simulink library "carnot"  (R2018b)
settings: Solver=VariableStepAuto  StartTime=0.0  StopTime=10.0  RelTol=1e-3
undefined symbols (not defined in the file or in its folder): A, A_earth, acol, Acol, ActPower1, ActPower2, ActPower3, Ad, Ad0, Ar, Au, Au0, Azimuth_Angle, B, Bd, Bd0, Br, Bu, Bu0, C, c1, c2, c3, c33, c4, c5, c6, CarnotCallbacks_Density, CarnotCallbacks_Enthalpy, CarnotCallbacks_Enthalpy2Temperature, CarnotCallbacks_Entropy, CarnotCallbacks_Evaporation_Enthalpy, CarnotCallbacks_GlobalMessageLevel, CarnotCallbacks_Grashof, CarnotCallbacks_Heat_Capacity, CarnotCallbacks_Kinematic_Viscosity, CarnotCallbacks_PMV_PPD, CarnotCallbacks_Prandtl, CarnotCallbacks_Saturation_Property, CarnotCallbacks_Saturation_Temperature, CarnotCallbacks_Saturation_Value_Water, CarnotCallbacks_Specific_Volume, CarnotCallbacks_Thermal_Conductivity, CarnotCallbacks_Vapour_Content, CarnotCallbacks_Vapour_Pressure, Cd, Cdl, Cr, Cu, Davies, Dd, DE_TRY2010_04_averageYear, delta_grd, density, DiameterLastPiece, dl, DPConstant, DPLinear, DPQuadratic, Dr ... (+59)
libraries: $bdroot x429, simulink x36, simulink_extras x12
(part 16 of 22)

== system carnot/Source/Cogeneration/microCHP_modulating ==
  THBreturn_load : Inport
  control : Inport  Port=2
  Bus Creator : BusCreator  Inputs=8
  Constant : Constant  Value=f_P_el
  Control_Unit : Subsystem
  Demux : Demux  Outputs=[1 1 1 1 1 1]
  Demux3 : Demux  Outputs=[6 14]
  Ground : Ground
  Heat_Capacity : $bdroot/Basic/Material_Properties/Heat_Capacity  VariantControl=CarlibClassic  INPUTARGUMENTS=state variables (classic)  DEBUGLEVEL=DEBUGLEVEL  MAXTOTALWARNINGS=inf  MAXCONSECUTIVEWARNINGS=inf  WRITETOFILE=0  FILENAME='errors.txt'
  Mux1 : Mux  Inputs=[1 1 1 1 1 1 14]
  Product : Product  Inputs=//*  SaturateOnIntegerOverflow=on  RndMeth=Zero  InputSameDT=on  OutDataTypeStr=Inherit: Same as first input
  Product1 : Product  Inputs=**  SaturateOnIntegerOverflow=on  RndMeth=Zero  InputSameDT=on  OutDataTypeStr=Inherit: Same as first input
  Product2 : Product  Inputs=**  SaturateOnIntegerOverflow=on  RndMeth=Zero  InputSameDT=on  OutDataTypeStr=Inherit: Same as first input
  Storage_Type_0 : $bdroot/Storage/Thermal/Storage_Type_0  t0=25  hgt=0.95493  stgtype=0  mpts=[1 2 3 4 5]  tini=[25 25 25 25 25]  PathName=fullfile(path_carnot('libsl'),'Storage','Thermal','Storage_Type_0','parameter_set')  FileName='<user defined>'  userPath=off  userParam=on  uwall=1  ubot=1  utop=1  axcond=1  volume=0.03  dia=0.2  standing=standing cylinder  nodes=5  mpoints=5  Tsensor=0.5  pipe1inlet=1  pipe1outlet=0  pipe1dia=0.03  heater1start=0.2  heater1end=0.25
  Sum : Sum  SaturateOnIntegerOverflow=on  InputSameDT=on  OutDataTypeStr=Inherit: Same as first input
  THB2THV : $bdroot/Toolbox/THB2THV
  THB2THV1 : $bdroot/Toolbox/THB2THV
  THV2THB : $bdroot/Toolbox/THV2THB
  THV2THB1 : $bdroot/Toolbox/THV2THB
  T_Sensor : $bdroot/Control/T_Sensor  tc=10  t0=20
  T_amb : Constant  Value=15
  Terminator : Terminator
  Terminator1 : Terminator
  energy and efficiency : Subsystem
  f_P_gas_lookup-table : Lookup_n-D  NumberOfTableDimensions=1  BreakpointsForDimension1=[1,2]  BreakpointsForDimension2=[44,80]  BreakpointsForDimension3=[1:2]  BreakpointsForDimension4=[1:2]  Table=[1.79 1.5]  InputSameDT=on
  measure_T : Subsystem  mask(temperature measurement sensor){tc=10, t0=25}
      mask prompts: tc "time constant of sensor [s]"; t0 "initial temperature [degree centigrade]"
      mask help: Measurement sensor for temperatures with first-oder hold. Temperature is in degree centigrade.
      mask init:
      | tc = 1/max(tc, 0.001);
      mask Help: eval('man (''measure_T'')')
      mask Display: plot(-18,0,30,20,[0 20],[0 0],[10 10 8 8 12 12 10],[0 8 8 17 17 8 8],[10 10 9 9 11 11 10 9],[15 10 10 9 9 10 9 10])
  measure_mdot : Subsystem  mask(massflow measurement sensor){}
      mask help: Measurement sensor for massflow in kg/s.
      mask Help: eval('man (''measure_mdot'')')
  pump_const : Subsystem  mask(constant pump){mdotmax=0.3, fluid_id=water, mix=0, dia=0.0157, power=100, p0=3e5}
      mask prompts: mdotmax "massflow rate [kg/s]"; fluid_id "fluid"; mix "percentage of fluid mix [0..1]"; dia "diameter at in- and outlet [m]"; power "electric power consumption [W]"; p0 "system pressure [Pa]"
      mask help: set constant massflow rate
      mask init:
      | mix = min(1, max(0, mix));
      | dia = max(0.001, dia);
      | p0 = max(p0, 1e5);
      mask Help: eval('man(''pump_const'')')
      mask TypeOptions fluid_id: water | air | cotton_oil | silicone_oil | water_glycol_mix
      mask Display: plot(0,0,100,100,[40,70,40,30,30,40,60,70,70,60,40],[70,50,30,40,60,70,70,60,40,30,30])
  return temperature raising facility : Subsystem  mask(return temperature raising facility){}
      mask help: A return setpoint temperature is calculated depending on heating power and flow setpoint temperature. The thermostatic mixer is located in the return flow of the CHP.
  scale_function : Subsystem
  zeroavoiding : Saturate  UpperLimit=inf  LowerLimit=1e-5
  THBflow_load : Outport
  data : Outport  Port=2
  wires:
  Ground/1 -> Storage_Type_0/3
  THBreturn_load/1 -> T_Sensor/1
  T_Sensor/2 -> Control_Unit/5(T_return_load)
  Storage_Type_0/2 -> Terminator1/1
  Demux/4 -> Mux1/4, Heat_Capacity/2  "p"
  Demux/1 -> Mux1/1  "ID"
  Demux/5 -> Mux1/5, Heat_Capacity/3
  Demux/6 -> Mux1/6, Heat_Capacity/4
  Demux/3 -> Mux1/3, zeroavoiding/1  "mdot"
  Sum/1 -> Mux1/2
  Demux3/1 -> Demux/1
  Demux3/2 -> Mux1/7
  Mux1/1 -> THV2THB1/1
  Product/1 -> Sum/2
  Demux/2 -> Heat_Capacity/1, Sum/1  "T"
  Heat_Capacity/1 -> Control_Unit/1(cp), Product/2
  measure_T/1(T) -> Control_Unit/3(T_flow)
  measure_mdot/2(mdot) -> Control_Unit/2(mdot_return)
  zeroavoiding/1 -> Product/1
  THB2THV1/1 -> pump_const/1(THVin)
  pump_const/1(THV) -> measure_T/1(THV_in)
  Control_Unit/1(control_CHP) -> Bus Creator/7, pump_const/2(control), energy and efficiency/1(control CHP)  "ControlActual"
  Control_Unit/2(P_th) -> Product/3, return temperature raising facility/2(P_th), energy and efficiency/2(P_th), Product2/1, scale_function/1(P_th), Product1/1
  scale_function/1(X_pth) -> f_P_gas_lookup-table/1
  Product2/1 -> energy and efficiency/4(P_el)
  f_P_gas_lookup-table/1 -> Product1/2
  Product1/1 -> energy and efficiency/3(P_gas)
  return temperature raising facility/1(THB_return) -> THB2THV/1
  measure_T/2(THV) -> THV2THB/1
  measure_mdot/1(THV) -> Demux3/1
  Constant/1 -> Product2/2
  energy and efficiency/1(Q_th) -> Bus Creator/1  "Q_th"
  energy and efficiency/2(Q_el) -> Bus Creator/2  "Q_el"
  energy and efficiency/3(Q_gas) -> Bus Creator/3  "Q_Gas"
  energy and efficiency/4(eta_th) -> Bus Creator/4  "eta_th"
  energy and efficiency/5(eta_el) -> Bus Creator/5  "eta_el"
  energy and efficiency/6(eta_sys) -> Bus Creator/6  "eta_sys"
  Bus Creator/1 -> data/1
  return temperature raising facility/2(THB_flow_load) -> THBflow_load/1
  T_Sensor/1 -> return temperature raising facility/3(THB_return_load)
  control/1 -> Bus Creator/8, Control_Unit/4(demand_control)  "ControlSetpoint"
  THB2THV/1 -> measure_mdot/1(THV_in)
  THV2THB/1 -> return temperature raising facility/1(THB_flow)
  THV2THB1/1 -> Storage_Type_0/2
  Storage_Type_0/3 -> THB2THV1/1
  T_amb/1 -> Storage_Type_0/1
  Storage_Type_0/1 -> Terminator/1

== system carnot/Source/Electric_Generator/Inverter ==
  note: power curtailment:
      | maximal possible power - actual power
  EB_DC : Inport
  P_max_set : Inport  Port=2
  1-D Lookup Table : Lookup_n-D  NumberOfTableDimensions=1  BreakpointsForDimension1=PstepsEta  Table=Eta  RndMeth=Simplest  InputSameDT=on
  Add : Sum  Inputs=+-
  Bus Assignment : BusAssignment  AssignedSignals=Frequency,Voltage1,ActPower1,Voltage2,ActPower2,Voltage3,ActPower3
  Bus Creator2 : BusCreator  Inputs=5
  Bus Selector : BusSelector  OutputSignals=ActPower1
  Compare To Zero : simulink/Logic and Bit Operations/Compare To Zero  relop===  OutDataTypeStr=boolean
  Demux : Demux  Outputs=3
  Frequency : Constant  Value=f
  Matrix1phase : Gain  Gain=[1 0 0]
  Matrix3phase : Gain  Gain=[1/3 1/3 1/3]
  MinMax : MinMax  Inputs=2
  NormialPower : Constant  Value=Pacnom
  Nphase : Constant  Value=nphase  mask{nphase=1-phase}
      mask prompts: nphase "Number of phases"
      mask TypeOptions nphase: 1-phase | 3-phase
  P_standby : Constant  Value=P_standby
  Product : Product
  Product1 : Product  Inputs=*/
  Product3 : Product
  Signal Conversion : SignalConversion  OverrideOpt=off
  Sum : Sum  Inputs=-+
  Switch : Switch  Criteria=u2 > Threshold  Threshold=1.5
  Voltage : Constant  Value=U
  basic_EB : $bdroot/Basic/Electric/basic_EB  eID=Power only  f=50  v1=230  p1=0  pf1=1  v2=230  p2=0  pf2=1  v3=230  p3=0  pf3=1
  limit_0_1 : Saturate  UpperLimit=inf  LowerLimit=0
  limit_Pacnom : Saturate  UpperLimit=Pacnom  LowerLimit=0
  only_positive : Saturate  UpperLimit=inf  LowerLimit=0
  EB_AC : Outport
  InvDat : Outport  Port=2
  wires:
  limit_Pacnom/1 -> MinMax/1, Sum/2
  limit_0_1/1 -> 1-D Lookup Table/1
  Nphase/1 -> Switch/2
  Matrix3phase/1 -> Switch/1
  Matrix1phase/1 -> Switch/3
  Switch/1 -> Demux/1
  Demux/1 -> Bus Assignment/4
  Demux/3 -> Bus Assignment/8
  Demux/2 -> Bus Assignment/6
  Voltage/1 -> Bus Assignment/3, Bus Assignment/5, Bus Assignment/7
  Frequency/1 -> Bus Assignment/2
  Bus Assignment/1 -> EB_AC/1
  basic_EB/1 -> Bus Assignment/1
  Add/1 -> Bus Creator2/1, Matrix1phase/1, Matrix3phase/1  "P_AC"
  Product3/1 -> Add/2
  P_standby/1 -> Product3/2
  Signal Conversion/1 -> Product3/1
  Compare To Zero/1 -> Signal Conversion/1
  1-D Lookup Table/1 -> Product/1
  Product/1 -> limit_Pacnom/1
  only_positive/1 -> MinMax/2
  NormialPower/1 -> Product1/2, Bus Creator2/4  "P_peak"
  Product1/1 -> limit_0_1/1
  Sum/1 -> Bus Creator2/5  "P_curtailment"
  Bus Creator2/1 -> InvDat/1  "InvDat"
  MinMax/1 -> Sum/1, Compare To Zero/1, Add/1  "P_AC"
  P_max_set/1 -> Bus Creator2/3, only_positive/1  "P_max_set"
  EB_DC/1 -> Bus Selector/1  "P_DC"
  Bus Selector/1 -> Product/2, Bus Creator2/2, Product1/1  "<ActPower1>"

== system carnot/Source/Electric_Generator/Inverter_SPI ==
  EB_PV : Inport
  EB_Load : Inport  Port=2
  PwrTarget : Inport  Port=3  Unit=W
  ac_charge_on : Inport  Port=4  Unit=W
  Bus Assignment : BusAssignment  AssignedSignals=ActPower1,ActPower2,ActPower3
  Bus Creator : BusCreator  Inputs=11
  Bus Selector : BusSelector  OutputSignals=ActPower1  OutputAsBus=on
  Bus Selector1 : BusSelector  OutputSignals=ActPower1  OutputAsBus=on
  Demux : Demux  Outputs=8
  Demux1 : Demux  Outputs=3
  Matrix1phase : Gain  Gain=[1 0 0]
  Matrix3phase : Gain  Gain=[1/3 1/3 1/3]
  Mux2 : Mux
  Nphase : Constant  Value=nphase  mask{nphase=3-phase}
      mask prompts: nphase "Number of phases"
      mask TypeOptions nphase: 1-phase | 3-phase
  S-Function : S-Function  FunctionName=Inverter_SPI  Parameters=soc0,cap_user,soc_min,soc_max,spi_data, inv_Ts  SFunctionDeploymentMode=off  EnableBusSupport=off  mask{spi_data=SpiData, soc0=soc0, soc_min=socMin, soc_max=socMax, inv_Ts=Tsample, cap_user=capUser}
      mask prompts: spi_data "SPI Parameters"; soc0 "initial state of charge"; soc_min "minimum  state of charge"; soc_max "maximum state of charge"; inv_Ts "sample Time"; cap_user "override battery capacity"
      mask init:
      | if isempty(spi_data)
      |    spi_data = [5;5;4;4;4;5;0;0;0;0;0;0;0;0;0;0;0;0;0;0;0;0;0;0;0.980000000000000;2;5;0;0;0;0;1;5;90] 
      | end
      | if isempty(soc0)
      |    soc0 = 0;
      | end
      | if isempty(soc_min)
      |    soc_min = 0;
      | end
      | if isempty(soc_max)
      |    soc_max = 0;
      | end
      | if isempty(inv_Ts)
      |    inv_Ts = 1;
      | end
      | if isempty(cap_user)
      |    cap_user = 0;
      | end
  Switch : Switch  Criteria=u2 > Threshold  Threshold=1.5
  gain : Gain  Gain=-1
  InvDat : Outport
  EB_AC : Outport  Port=2
  wires:
  EB_PV/1 -> Bus Selector/1  "P_DC"
  Demux/8 -> Bus Creator/8  "Ebat"
  Demux/2 -> Bus Creator/2  "Ppv2ac"
  Mux2/1 -> S-Function/1
  Demux/3 -> Bus Creator/3  "Pbat2ac"
  PwrTarget/1 -> Mux2/3, Bus Creator/9  "PowerTarget"
  Demux/6 -> Bus Creator/6  "Pbat"
  Demux/4 -> Bus Creator/4  "Pac2bat"
  Demux/7 -> Bus Creator/7  "SOC"
  gain/1 -> Mux2/2  "Pac"
  Demux/5 -> Bus Creator/5  "Ppv2bat"
  Bus Creator/1 -> InvDat/1
  Bus Selector/1 -> Bus Creator/10, Mux2/1  "Ppv"
  Demux/1 -> Bus Creator/1, Matrix3phase/1, Matrix1phase/1  "Ppvbs"
  S-Function/1 -> Demux/1
  EB_Load/1 -> Bus Selector1/1, Bus Assignment/1  "P_AC"
  Demux1/1 -> Bus Assignment/2
  Demux1/2 -> Bus Assignment/3
  Bus Assignment/1 -> EB_AC/1
  Demux1/3 -> Bus Assignment/4
  Nphase/1 -> Switch/2
  Matrix3phase/1 -> Switch/1
  Matrix1phase/1 -> Switch/3
  Switch/1 -> Demux1/1
  Bus Selector1/1 -> gain/1, Bus Creator/11  "Pload"
  ac_charge_on/1 -> Mux2/4

== system carnot/Source/Electric_Generator/PV_Generator ==
  WDB : Inport
  position : Inport  Port=2
  1/(1000W/m²) : Gain  Gain=1/1000
  Bus Creator : BusCreator  Inputs=4
  Bus Selector1 : BusSelector  OutputSignals=Temperature_Ambient
  EBCreator : $bdroot/Basic/Electric/EBCreator  Inport_ID=off  Inport_f=off  Inport_v1=off  Inport_p1=on  Inport_pf1=off  Inport_v2=off  Inport_p2=off  Inport_pf2=off  Inport_v3=off  Inport_p3=off  Inport_pf3=off  ID=1  f=0  v1=0  p1=1e5  pf1=1  v2=0  p2=0  pf2=0  v3=0  p3=0  pf3=0  Annotation_ID=off  Annotation_f=off  Annotation_v1=off  Annotation_p1=off  Annotation_pf1=off  Annotation_v2=off  Annotation_p2=off  Annotation_pf2=off  Annotation_v3=off  Annotation_p3=off  Annotation_pf3=off
  IAM_Table1 : $bdroot/Source/Solar_Thermal/IncidenceAngleModifier/IAM_Table  fta=1  angle=[0:5:90]  Kb="[1.0000    1.0000    0.9999    0.9996    0.9991    0.9982    0.9965  0.9935    0.9886    0.9807    0.9678    0.9473    0.9148    0.8638   0.7846    0.6644    0.4907    0.2599    0.0000]"  Kd=0.915
  Product : Product  RndMeth=Zero
  Radiation_on_Inclined_Surface : $bdroot/Weather/Radiation_on_Inclined_Surface  sky=Hay-Davies  reflect=0.2
  Sum : Sum  Inputs=-+
  T module : Sum  Inputs=2
  T0 : Constant  Value=25
  Wp : Constant  Value=Wp
  Wp_act : Sum
  delta_Wp : Product  RndMeth=Zero
  delta_Wp/K : Gain  Gain=delta_Wp_K
  factor for generator : Gain  Gain=fgen
  overheating 40K@1000W/m2 : Gain  Gain=40
  EB_power : Outport
  PVdat : Outport  Port=2
  wires:
  EBCreator/1 -> EB_power/1
  Bus Creator/1 -> PVdat/1
  delta_Wp/1 -> Wp_act/1
  Wp/1 -> delta_Wp/2, Bus Creator/4, Wp_act/2  "P_peak_PV"
  Bus Selector1/1 -> T module/2  "<Temperature_Ambient>"
  overheating 40K@1000W/m2/1 -> T module/1
  Sum/1 -> delta_Wp/K/1
  T0/1 -> Sum/2
  IAM_Table1/1 -> 1/(1000W/m²)/1
  T module/1 -> Bus Creator/3, Sum/1  "Tcell"
  Wp_act/1 -> Product/2
  1/(1000W/m²)/1 -> overheating 40K@1000W/m2/1, Product/1
  Product/1 -> factor for generator/1
  delta_Wp/K/1 -> delta_Wp/1
  factor for generator/1 -> Bus Creator/1, EBCreator/1  "P_DC"
  WDB/1 -> Bus Selector1/1, Radiation_on_Inclined_Surface/1
  Radiation_on_Inclined_Surface/1 -> IAM_Table1/1
  position/1 -> Radiation_on_Inclined_Surface/2
  IAM_Table1/2 -> Bus Creator/2  "SolarRadiaton_global_surface"

== system carnot/Source/Energy/Fuel ==
  Bus Creator : BusCreator  Inputs=13
  Demux : Demux  Outputs=6
  airdemand : Constant  Value=stoichAir
  enthalpy : Constant  Value=combustion_enthalpy
  fuel_type : Constant  Value=ft
  mass : Constant  Value=massfraction
  pressure : Constant  Value=Pressure
  price : Constant  Value=price
  tc : Constant  Value=Tcondensation
  temperature : Constant  Value=Temperature
  fuel : Outport
  wires:
  mass/1 -> Demux/1
  airdemand/1 -> Bus Creator/3  "Stoichiometric_Air_Demand"
  Demux/6 -> Bus Creator/13  "MassFraction_H2O"
  pressure/1 -> Bus Creator/4  "Pressure"
  price/1 -> Bus Creator/7  "Price"
  Demux/3 -> Bus Creator/10  "MassFraction_O"
  enthalpy/1 -> Bus Creator/5  "h_Vector"
  Demux/1 -> Bus Creator/8  "MassFraction_H"
  Bus Creator/1 -> fuel/1
  Demux/4 -> Bus Creator/11  "MassFraction_S"
  Demux/5 -> Bus Creator/12  "MassFraction_N"
  tc/1 -> Bus Creator/6  "T_h_Vector"
  fuel_type/1 -> Bus Creator/1  "Fuel_ID"
  Demux/2 -> Bus Creator/9  "MassFraction_C"
  temperature/1 -> Bus Creator/2  "Temperature"

== system carnot/Source/Heat_Exchanger/Floorheating_TABS ==
  note: source: Koschenz, M.; Lehmann, B.: Thermoaktive Bauteilsysteme tabs. EMPA, Dübendorf, 2000. ISBN 3-905594-19-6
  T(P) : Inport
  THBin : Inport  Port=2
  Bus Assignment : BusAssignment  AssignedSignals=Temperature
  Bus Selector : BusSelector  OutputSignals=Temperature,MassFlow,Pressure,FluidType,FluidMix
  Demux2 : Demux  Outputs=2
  Mux2 : Mux  Inputs=6
  S-Function : S-Function  FunctionName=tabs  Parameters=d d1 d_pipe dr dx l lambda_r lambda_b  SFunctionDeploymentMode=off  EnableBusSupport=off
  power : Outport
  THBout : Outport  Port=2  InitialOutput=0
  wires:
  T(P)/1 -> Mux2/6
  THBin/1 -> Bus Assignment/1, Bus Selector/1
  Bus Selector/4 -> Mux2/4  "<FluidType>"
  Bus Selector/3 -> Mux2/3  "<Pressure>"
  Bus Selector/2 -> Mux2/2  "<MassFlow>"
  Bus Selector/5 -> Mux2/5  "<FluidMix>"
  Bus Selector/1 -> Mux2/1  "<Temperature>"
  Mux2/1 -> S-Function/1
  S-Function/1 -> Demux2/1
  Demux2/2 -> Bus Assignment/2  "Temperature"
  Demux2/1 -> power/1
  Bus Assignment/1 -> THBout/1

== system carnot/Source/Heat_Exchanger/HeatExchanger ==
  Tamb : Inport
  THB_pri : Inport  Port=2
  THB_sec : Inport  Port=3
  Bus Assignment : BusAssignment  AssignedSignals=Temperature
  Bus Assignment1 : BusAssignment  AssignedSignals=Temperature
  Bus Selector : BusSelector  OutputSignals=Temperature,MassFlow,Pressure,FluidType,FluidMix  OutputAsBus=on
  Bus Selector1 : BusSelector  OutputSignals=Temperature,MassFlow,Pressure,FluidType,FluidMix  OutputAsBus=on
  Pressure_Drop_Fix : $bdroot/Basic/Pressure_Drop/Pressure_Drop_Fix  con=0  lin=linh  qua=quah
  Pressure_Drop_Fix1 : $bdroot/Basic/Pressure_Drop/Pressure_Drop_Fix  con=0  lin=linc  qua=quac
  S-Function : S-Function  FunctionName=heatexch  Parameters=flowtype, ua0, uahot(1), uahot(2), uacold(1), uacold(2), ualoss, cap, t0  SFunctionDeploymentMode=off  EnableBusSupport=off
  Terminator : Terminator
  THBpri : Outport
  THBsec : Outport  Port=2
  wires:
  Pressure_Drop_Fix1/1 -> THBsec/1
  Pressure_Drop_Fix/1 -> THBpri/1
  Bus Assignment1/1 -> Pressure_Drop_Fix1/1
  S-Function/2 -> Bus Assignment1/2
  Bus Assignment/1 -> Pressure_Drop_Fix/1
  S-Function/1 -> Bus Assignment/2
  Bus Selector1/1 -> S-Function/3
  THB_sec/1 -> Bus Assignment1/1, Bus Selector1/1
  THB_pri/1 -> Bus Assignment/1, Bus Selector/1
  S-Function/3 -> Terminator/1
  Bus Selector/1 -> S-Function/2
  Tamb/1 -> S-Function/1

== system carnot/Source/Heat_Exchanger/Radiator ==
  Troom : Inport
  THBin : Inport  Port=2
  Radiator_basic : $bdroot/Basic/Thermal_Models/Radiator_basic  pnomEN=pnom  dtnomEN=dtnom  expo=expo  mcp=mcap  tini=tini
  pressdrop_fix_THB : $bdroot/Basic/Pressure_Drop/Pressure_Drop_Fix  con=0  lin=lin  qua=qua
  Qdot : Outport
  THBout : Outport  Port=2
  wires:
  pressdrop_fix_THB/1 -> THBout/1
  Radiator_basic/1 -> pressdrop_fix_THB/1
  THBin/1 -> Radiator_basic/1
  Troom/1 -> Radiator_basic/2
  Radiator_basic/2 -> Qdot/1

== system carnot/Source/Heat_Exchanger/Radiator_AIV ==
  AIV : Inport
  THB_in : Inport  Port=2
  Ground : Ground
  Ground1 : Ground
  Ground2 : Ground
  Matrix Gain : Gain  Gain=[co; ra]  Multiplication=Matrix(K*u)  SaturateOnIntegerOverflow=on  OutDataTypeStr=Inherit: Same as input  ParamDataTypeStr=Inherit: Same as input
  Mux2 : Mux  Inputs=[4 1 1 2 5]
  Radiator : $bdroot/Source/Heat_Exchanger/Radiator  pnom=pnom  dtnom=dtnom  expo=expo  mcap=mcap  tini=tini  lin=lin  qua=qua
  Troom : Subsystem
  S : Outport
  THB_out : Outport  Port=2
  wires:
  Ground/1 -> Mux2/1
  Ground2/1 -> Mux2/3
  Ground1/1 -> Mux2/5
  Mux2/1 -> S/1
  Matrix Gain/1 -> Mux2/4  "[Qdotc Qdotr]"
  Radiator/1 -> Matrix Gain/1, Mux2/2
  AIV/1 -> Troom/1("[AIV]")
  Troom/1(Troom) -> Radiator/1
  THB_in/1 -> Radiator/2
  Radiator/2 -> THB_out/1

== system carnot/Source/Heat_Exchanger/THB_P_adapter ==
  note: (°C)
  T(P) : Inport
  THBin : Inport  Port=2
  -1 : Gain  Gain=-1  SaturateOnIntegerOverflow=on  OutDataTypeStr=Inherit: Same as input  ParamDataTypeStr=Inherit: Same as input
  Bus Assignment : BusAssignment  AssignedSignals=Temperature
  Bus Selector : BusSelector  OutputSignals=Temperature,MassFlow
  Heat_Capacity : $bdroot/Basic/Material_Properties/Heat_Capacity  VariantControl=CarlibClassic  INPUTARGUMENTS=THB  DEBUGLEVEL=DEBUGLEVEL  MAXTOTALWARNINGS=inf  MAXCONSECUTIVEWARNINGS=inf  WRITETOFILE=0  FILENAME='errors.txt'
  Integrator : Integrator  InitialCondition=t0
  Product1 : Product  Inputs=3  SaturateOnIntegerOverflow=on  InputSameDT=on  OutDataTypeStr=Inherit: Same as first input
  Product2 : Product  Inputs=/*  SaturateOnIntegerOverflow=on  InputSameDT=on  OutDataTypeStr=Inherit: Same as first input
  Sum1 : Sum  Inputs=-+  SaturateOnIntegerOverflow=on  InputSameDT=on  OutDataTypeStr=Inherit: Same as first input
  Sum2 : Sum  SaturateOnIntegerOverflow=on  InputSameDT=on  OutDataTypeStr=Inherit: Same as first input
  Sum3 : Sum  Inputs=+-  SaturateOnIntegerOverflow=on  InputSameDT=on  OutDataTypeStr=Inherit: Same as first input
  heat transfer : Gain  Gain=ua  SaturateOnIntegerOverflow=on  OutDataTypeStr=Inherit: Same as input  ParamDataTypeStr=Inherit: Same as input
  mass : Gain  Gain=mass  SaturateOnIntegerOverflow=on  OutDataTypeStr=Inherit: Same as input  ParamDataTypeStr=Inherit: Same as input
  power : Outport
  THB : Outport  Port=2
  wires:
  Bus Assignment/1 -> THB/1
  Sum3/1 -> Product1/1
  Bus Selector/2 -> Product1/2  "<MassFlow>"
  Product1/1 -> Sum2/1
  Heat_Capacity/1 -> Product1/3, mass/1
  Bus Selector/1 -> Sum3/1  "<Temperature>"
  Sum1/1 -> heat transfer/1
  T(P)/1 -> Sum1/2  "Tnode"
  Integrator/1 -> Sum1/1, Bus Assignment/2, Sum3/2  "Twater"
  mass/1 -> Product2/1
  Product2/1 -> Integrator/1
  Sum2/1 -> Product2/2
  -1/1 -> power/1
  heat transfer/1 -> Sum2/2, -1/1  "Qdot"
  THBin/1 -> Heat_Capacity/1, Bus Assignment/1, Bus Selector/1

== system carnot/Source/Heat_Exchanger/VDIHeatExchanger ==
  Tamb : Inport
  THB_in_source : Inport  Port=2
  THB_in_load : Inport  Port=3
  Bus Assignment : BusAssignment  AssignedSignals=Temperature
  Bus Assignment1 : BusAssignment  AssignedSignals=Temperature
  Bus Selector : BusSelector  OutputSignals=Temperature,MassFlow,Pressure,FluidType,FluidMix  OutputAsBus=on
  Bus Selector1 : BusSelector  OutputSignals=Temperature,MassFlow,Pressure,FluidType,FluidMix  OutputAsBus=on
  Pressure_Drop_Fix : $bdroot/Basic/Pressure_Drop/Pressure_Drop_Fix  con=0  lin=linh  qua=quah
  Pressure_Drop_Fix1 : $bdroot/Basic/Pressure_Drop/Pressure_Drop_Fix  con=0  lin=linc  qua=quac
  S-Function : S-Function  FunctionName=VDIheatexch  Parameters=flowtype, ua0, uahot(1), uahot(2), uacold(1), uacold(2), ualoss, cap, t0,a,b,c,d  SFunctionDeploymentMode=off  EnableBusSupport=off
  Terminator : Terminator
  Terminator1 : Terminator
  THB_out_source : Outport
  THB_out_load : Outport  Port=2
  wires:
  S-Function/4 -> Terminator1/1
  Pressure_Drop_Fix1/1 -> THB_out_load/1
  Pressure_Drop_Fix/1 -> THB_out_source/1
  Bus Assignment1/1 -> Pressure_Drop_Fix1/1
  S-Function/2 -> Bus Assignment1/2
  Bus Assignment/1 -> Pressure_Drop_Fix/1
  S-Function/1 -> Bus Assignment/2
  Bus Selector1/1 -> S-Function/3
  THB_in_load/1 -> Bus Assignment1/1, Bus Selector1/1
  THB_in_source/1 -> Bus Assignment/1, Bus Selector/1
  S-Function/3 -> Terminator/1
  Bus Selector/1 -> S-Function/2
  Tamb/1 -> S-Function/1

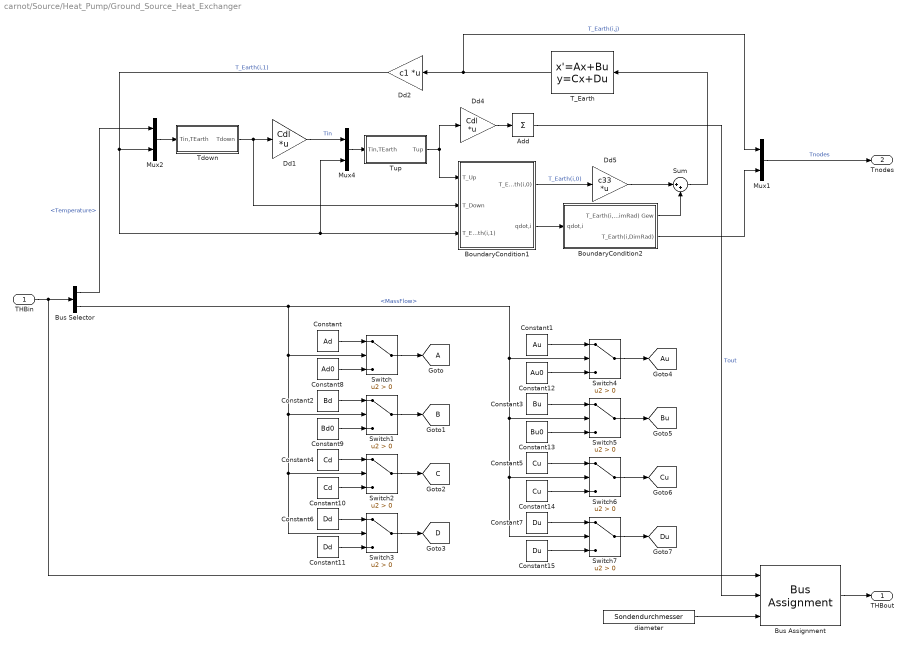
== system carnot/Source/Heat_Pump/Ground_Source_Heat_Exchanger ==
  THBin : Inport
  Add : Sum  Inputs=1
  BoundaryCondition1 : Subsystem
  BoundaryCondition2 : Subsystem
  Bus Assignment : BusAssignment  AssignedSignals=Temperature,DiameterLastPiece
  Bus Selector : BusSelector  OutputSignals=Temperature,MassFlow
  Constant : Constant  Value=Ad
  Constant1 : Constant  Value=Au
  Constant10 : Constant  Value=Cd
  Constant11 : Constant  Value=Dd
  Constant12 : Constant  Value=Au0
  Constant13 : Constant  Value=Bu0
  Constant14 : Constant  Value=Cu
  Constant15 : Constant  Value=Du
  Constant2 : Constant  Value=Bd
  Constant3 : Constant  Value=Bu
  Constant4 : Constant  Value=Cd
  Constant5 : Constant  Value=Cu
  Constant6 : Constant  Value=Dd
  Constant7 : Constant  Value=Du
  Constant8 : Constant  Value=Ad0
  Constant9 : Constant  Value=Bd0
  Dd1 : Gain  Gain=Cdl  Multiplication=Matrix(K*u)  SaturateOnIntegerOverflow=on  OutDataTypeStr=Inherit: Same as input  ParamDataTypeStr=Inherit: Same as input
  Dd2 : Gain  Gain=c1  Multiplication=Matrix(K*u)  SaturateOnIntegerOverflow=on  OutDataTypeStr=Inherit: Same as input  ParamDataTypeStr=Inherit: Same as input
  Dd4 : Gain  Gain=Cdl  Multiplication=Matrix(K*u)  SaturateOnIntegerOverflow=on  OutDataTypeStr=Inherit: Same as input  ParamDataTypeStr=Inherit: Same as input
  Dd5 : Gain  Gain=c33  Multiplication=Matrix(K*u)  SaturateOnIntegerOverflow=on  OutDataTypeStr=Inherit: Same as input  ParamDataTypeStr=Inherit: Same as input
  Mux1 : Mux  Inputs=2
  Mux2 : Mux  Inputs=2
  Mux4 : Mux  Inputs=2
  Sum : Sum  Inputs=|++  SaturateOnIntegerOverflow=on  InputSameDT=on  OutDataTypeStr=Inherit: Same as first input
  Switch{,1..7} (8 alike) : Switch  Criteria=u2 > Threshold
  T_Earth : StateSpace  A=Ar  B=Br  C=Cr  D=Dr  InitialCondition=Tearth_anf(:)
  Tdown : Subsystem
  Tup : Subsystem
  diameter : Constant  Value=Sondendurchmesser
  THBout : Outport
  Tnodes : Outport  Port=2
  tag scope: A=global, Au=global, B=global, Bu=global, C=global, Cu=global, D=global, Du=global
  wires:
  BoundaryCondition1/2(qdot,i) -> BoundaryCondition2/1(qdot,i)
  Mux1/1 -> Tnodes/1  "Tnodes"
  Add/1 -> Bus Assignment/2  "Tout"
  Dd4/1 -> Add/1
  Bus Assignment/1 -> THBout/1
  diameter/1 -> Bus Assignment/3
  THBin/1 -> Bus Assignment/1, Bus Selector/1
  BoundaryCondition2/2(T_Earth(i,DimRad)) -> Mux1/2
  Dd2/1 -> Mux2/2, BoundaryCondition1/3(T_Earth(i,1)), Mux4/2  "T_Earth(i,1)"
  BoundaryCondition1/1(T_Earth(i,0)) -> Dd5/1  "T_Earth(i,0)"
  Sum/1 -> T_Earth/1
  BoundaryCondition2/1(T_Earth(i,DimRad) Gew) -> Sum/2
  Dd5/1 -> Sum/1
  Tup/1(Tup) -> BoundaryCondition1/1(T_Up), Dd4/1
  T_Earth/1 -> Mux1/1, Dd2/1  "T_Earth(i,j)"
  Dd1/1 -> Mux4/1  "Tin"
  Mux4/1 -> Tup/1(Tin,TEarth)
  Mux2/1 -> Tdown/1(Tin,TEarth)
  Tdown/1(Tdown) -> BoundaryCondition1/2(T_Down), Dd1/1
  Switch/1 -> [A]
  Constant8/1 -> Switch/3
  Switch1/1 -> [B]
  Constant/1 -> Switch/1
  Constant2/1 -> Switch1/1
  Constant9/1 -> Switch1/3
  Switch2/1 -> [C]
  Constant4/1 -> Switch2/1
  Switch3/1 -> [D]
  Constant10/1 -> Switch2/3
  Constant11/1 -> Switch3/3
  Constant6/1 -> Switch3/1
  Constant1/1 -> Switch4/1
  Constant3/1 -> Switch5/1
  Constant5/1 -> Switch6/1
  Constant7/1 -> Switch7/1
  Switch7/1 -> [Du]
  Switch6/1 -> [Cu]
  Switch5/1 -> [Bu]
  Switch4/1 -> [Au]
  Constant15/1 -> Switch7/3
  Constant14/1 -> Switch6/3
  Constant13/1 -> Switch5/3
  Constant12/1 -> Switch4/3
  Bus Selector/2 -> Switch2/2, Switch3/2, Switch1/2, Switch/2, Switch6/2, Switch7/2, Switch5/2, Switch4/2  "<MassFlow>"
  Bus Selector/1 -> Mux2/1  "<Temperature>"

== system carnot/Source/Heat_Pump/HeatPump ==
  note: output range is 0 to 1
  note: set values below QdotMin to Zero
  THBsource : Inport
  THB_r : Inport  Port=2
  Tamb : Inport  Port=3
  Ctrl : Inport  Port=4
  Bus Assignment1 : BusAssignment  AssignedSignals=THBout_cold.Pressure,THBout_cold.DPConstant,THBout_cold.DPLinear,THBout_cold.DPQuadratic,THBout_hot.Pressure,THBout_hot.DPConstant,THBout_hot.DPLinear,THBout_hot.DPQuadratic
  Bus Creator1 : BusCreator  Inputs=9
  Bus Selector : BusSelector  OutputSignals=Pressure,DPConstant,DPLinear,DPQuadratic
  Bus Selector1 : BusSelector  OutputSignals=Pressure,DPConstant,DPLinear,DPQuadratic
  Bus Selector2 : BusSelector  OutputSignals=THBin_cold,THBout_cold,Qdot_cold,THBin_hot,THBout_hot,Qdot_hot,Pelec
  Constant : Constant  Value=0
  HeatPump_basic : $bdroot/Basic/Thermal_Models/HeatPump_basic  K=K  caph=caph  capc=capc  UA=UA
  Pressure_Drop_Cold : $bdroot/Basic/Pressure_Drop/Pressure_Drop_Fix  con=0  lin=linc  qua=quac
  Pressure_Drop_Hot : $bdroot/Basic/Pressure_Drop/Pressure_Drop_Fix  con=0  lin=linh  qua=quah
  Saturation : Saturate  UpperLimit=1  LowerLimit=0
  Switch : Switch  Threshold=relQdotMin
  THB_source : Outport
  THB_s : Outport  Port=2
  HPdat : Outport  Port=3
  wires:
  Bus Selector2/1 -> Bus Creator1/1  "<THBin_cold>"
  Saturation/1 -> HeatPump_basic/4, Bus Creator1/8  "ControlActual"
  Bus Selector2/2 -> Bus Creator1/2  "<THBout_cold>"
  Ctrl/1 -> Switch/2, Switch/1, Bus Creator1/9  "ControlSetpoint"
  Bus Selector2/6 -> Bus Creator1/6  "<Qdot_hot>"
  Bus Selector2/3 -> Bus Creator1/3  "<Qdot_cold>"
  Bus Assignment1/1 -> Bus Selector2/1
  Bus Selector2/5 -> Bus Creator1/5  "<THBout_hot>"
  Bus Creator1/1 -> HPdat/1
  Bus Selector2/4 -> Bus Creator1/4  "<THBin_hot>"
  Bus Selector2/7 -> Bus Creator1/7  "<Pelec>"
  Switch/1 -> Saturation/1
  Constant/1 -> Switch/3
  Pressure_Drop_Hot/1 -> THB_s/1, Bus Selector1/1  "THB_s"
  HeatPump_basic/2 -> Pressure_Drop_Hot/1
  THBsource/1 -> HeatPump_basic/1
  THB_r/1 -> HeatPump_basic/2
  Tamb/1 -> HeatPump_basic/3
  HeatPump_basic/1 -> Pressure_Drop_Cold/1
  Pressure_Drop_Cold/1 -> THB_source/1, Bus Selector/1  "THBsource"
  HeatPump_basic/3 -> Bus Assignment1/1  "HPdat"
  Bus Selector/1 -> Bus Assignment1/2  "<Pressure>"
  Bus Selector/2 -> Bus Assignment1/3  "<DPConstant>"
  Bus Selector/3 -> Bus Assignment1/4  "<DPLinear>"
  Bus Selector/4 -> Bus Assignment1/5  "<DPQuadratic>"
  Bus Selector1/1 -> Bus Assignment1/6  "<Pressure>"
  Bus Selector1/2 -> Bus Assignment1/7  "<DPConstant>"
  Bus Selector1/3 -> Bus Assignment1/8  "<DPLinear>"
  Bus Selector1/4 -> Bus Assignment1/9  "<DPQuadratic>"

== system carnot/Source/Simple/Constant_EB ==
  basic_EB : $bdroot/Basic/Electric/basic_EB  eID=Power only  f=f  v1=v1  p1=p1  pf1=pf1  v2=v2  p2=p2  pf2=pf2  v3=v3  p3=p3  pf3=pf3
  EB_out : Outport
  wires:
  basic_EB/1 -> EB_out/1

== system carnot/Source/Simple/Constant_THB ==
  basic_THB : $bdroot/Basic/Hydraulics/basic_THB  t=t  mdot=mdot  p=p  ID=No Pressure Drop  fluid=Water  mix=mix  mix2=mix2  mix3=mix3  dia=dia  hgt=hgt
  THB_out : Outport
  wires:
  basic_THB/1 -> THB_out/1

== system carnot/Source/Simple/EB_set_power ==
  EB_in : Inport
  act_power : Inport  Port=2
  Bus Assignment : BusAssignment  AssignedSignals=ActPower1,ActPower2,ActPower3
  Demux : Demux  Outputs=[1,1,1]
  EB : Outport
  wires:
  EB_in/1 -> Bus Assignment/1
  Bus Assignment/1 -> EB/1
  Demux/1 -> Bus Assignment/2
  Demux/2 -> Bus Assignment/3
  Demux/3 -> Bus Assignment/4
  act_power/1 -> Demux/1

== system carnot/Source/Simple/EB_set_voltage ==
  EB_in : Inport
  voltage : Inport  Port=2
  Bus Assignment : BusAssignment  AssignedSignals=Voltage1,Voltage2,Voltage3
  Demux : Demux  Outputs=[1,1,1]
  EB : Outport
  wires:
  voltage/1 -> Demux/1
  Demux/3 -> Bus Assignment/4
  Demux/2 -> Bus Assignment/3
  Demux/1 -> Bus Assignment/2
  Bus Assignment/1 -> EB/1
  EB_in/1 -> Bus Assignment/1

== system carnot/Source/Simple/THB_fixed_T ==
  THB_in : Inport
  THB_set_T : $bdroot/Source/Simple/THB_set_T
  Temperature : Constant  Value=t
  THB : Outport
  wires:
  THB_set_T/1 -> THB/1
  THB_in/1 -> THB_set_T/1
  Temperature/1 -> THB_set_T/2

== system carnot/Source/Simple/THB_fixed_mdot ==
  THB_in : Inport
  THB_set_mdot : $bdroot/Source/Simple/THB_set_mdot
  mdot : Constant  Value=m
  THB : Outport
  wires:
  mdot/1 -> THB_set_mdot/2
  THB_in/1 -> THB_set_mdot/1
  THB_set_mdot/1 -> THB/1

== system carnot/Source/Simple/THB_set_T ==
  THB_in : Inport
  T : Inport  Port=2
  Bus Assignment : BusAssignment  AssignedSignals=Temperature
  THB : Outport
  wires:
  THB_in/1 -> Bus Assignment/1
  Bus Assignment/1 -> THB/1
  T/1 -> Bus Assignment/2

== system carnot/Source/Simple/THB_set_mdot ==
  THB_in : Inport
  mdot : Inport  Port=2
  Bus Assignment : BusAssignment  AssignedSignals=MassFlow
  THB : Outport
  wires:
  mdot/1 -> Bus Assignment/2
  Bus Assignment/1 -> THB/1
  THB_in/1 -> Bus Assignment/1

== system carnot/Source/Simple/create_EB ==
  voltage : Inport
  act_power : Inport  Port=2
  basic_create_EB : $bdroot/Basic/Electric/basic_create_EB  eID=Power only  f=f  pf1=pf1  pf2=pf2  pf3=pf3
  EB : Outport
  wires:
  basic_create_EB/1 -> EB/1
  act_power/1 -> basic_create_EB/2
  voltage/1 -> basic_create_EB/1

== system carnot/Source/Simple/create_THB ==
  mdot : Inport
  T : Inport  Port=2
  basic_create_THB : $bdroot/Basic/Hydraulics/basic_create_THB  p=p  fluid=Water  mix=mix  mix2=mix2  mix3=mix3  dia=dia  hgt=hgt  mID=No Pressure Drop
  THB : Outport
  wires:
  mdot/1 -> basic_create_THB/1
  basic_create_THB/1 -> THB/1
  T/1 -> basic_create_THB/2

== system carnot/Source/Solar_Thermal/Collector_1xN ==
  WDB : Inport
  position : Inport  Port=2
  THB_r : Inport  Port=3
  Bus Assignment : BusAssignment  AssignedSignals=Temperature
  Bus Selector : BusSelector  OutputSignals=Temperature_Ambient,Wind_Speed,Temperature_Sky_Radiation
  Bus Selector1 : BusSelector  OutputSignals=Temperature,MassFlow
  Bus Selector2 : BusSelector  OutputSignals=Pressure,FluidType,FluidMix  OutputAsBus=on
  Mux2 : Mux  Inputs=5
  PowerMeter : $bdroot/Control/PowerMeter
  Pressure_Drop_Collector : $bdroot/Basic/Pressure_Drop/Pressure_Drop_Collector  len=len  lin=lin  qua=qua
  Radiation_on_Inclined_Surface : $bdroot/Weather/Radiation_on_Inclined_Surface  sky=Perez 1990  reflect=0.2
  Theoretical_Collector_Optics : $bdroot/Source/Solar_Thermal/IncidenceAngleModifier/Theoretical_Collector_Optics  FTA=eta0  ncover=1  refin=1.525  d=0.004  ext=4
  const : Constant  Value=acol
  create_Cdat : Subsystem
  universal collector : S-Function  FunctionName=unicol  Parameters=acol, u1, u2, u3, uwind, c_col, tini, nodes  SFunctionDeploymentMode=off  EnableBusSupport=off
  Cdat : Outport
  THB_s : Outport  Port=2
  wires:
  Bus Assignment/1 -> Pressure_Drop_Collector/2
  universal collector/3 -> Pressure_Drop_Collector/1  "Tnodes"
  PowerMeter/1 -> create_Cdat/4(Qdot)
  Bus Selector2/1 -> universal collector/4
  Bus Selector1/2 -> universal collector/3  "<MassFlow>"
  Bus Selector1/1 -> universal collector/2  "<Temperature>"
  Mux2/1 -> universal collector/1
  Bus Selector/3 -> Mux2/5  "<Temperature_Sky_Radiation>"
  Theoretical_Collector_Optics/2 -> Mux2/2
  Theoretical_Collector_Optics/1 -> Mux2/1
  Bus Selector/1 -> Mux2/3  "<Temperature_Ambient>"
  Bus Selector/2 -> Mux2/4  "<Wind_Speed>"
  Pressure_Drop_Collector/1 -> PowerMeter/1, create_Cdat/3(THBout), THB_s/1  "THB_s"
  universal collector/1 -> Bus Assignment/2
  universal collector/2 -> create_Cdat/5(Tmean)
  Radiation_on_Inclined_Surface/1 -> Bus Selector/1, Theoretical_Collector_Optics/1, create_Cdat/6(WDB)
  position/1 -> Pressure_Drop_Collector/3, Radiation_on_Inclined_Surface/2
  WDB/1 -> Radiation_on_Inclined_Surface/1
  THB_r/1 -> Bus Selector2/1, PowerMeter/2, create_Cdat/2(THBin), Bus Assignment/1, Bus Selector1/1
  const/1 -> create_Cdat/1(acol)
  create_Cdat/1(data_c) -> Cdat/1  "Cdat"

== system carnot/Source/Solar_Thermal/Collector_Unglazed ==
  WDB : Inport
  position : Inport  Port=2
  THBr : Inport  Port=3
  Bus Assignment : BusAssignment  AssignedSignals=MassFlow
  Bus Assignment1 : BusAssignment  AssignedSignals=MassFlow
  Bus Assignment2 : BusAssignment  AssignedSignals=Acol,Qdot,THBin.MassFlow,THBout.MassFlow
  Bus Selector : BusSelector  OutputSignals=MassFlow
  Bus Selector1 : BusSelector  OutputSignals=Acol,Qdot
  Collector_Unglazed : Subsystem  mask(Unglazed flat plate collector){acol=acol, len=len, fta=fta, e_sky=eps, uc0=u0c, uc1=u1c, uc0loss=u0l, uc1loss=u1l, uc0gain=u0g, uc1gain=u1g, uc1eta0=u1e, hi=hi, c_abs=capa, c_fl=capf, lin=dplin, qua=dpqua, tini=tini, nodes=nodes}
      mask prompts: acol "collector surface (aperture) in [m²]"; len "length between inlet and outlet [m]"; fta "absorption coefficient of the absorber [-]"; e_sky "e thermal emissivity of the absorber (0..1)"; uc0 "U0C heat transfer for condensation [W/(m²*K)]"; uc1 "U1C wind dependent heat transfer for condensation [W/(m²*K*m/s)]"; uc0loss "U0L heat transfer for losses [W/(m²*K)]"; uc1loss "U1L wind dependent heat transfer for losses [W/(m²*K*m/s)]"; uc0gain "U0G heat transfer for gains [W/(m²*K)]"; uc1gain "U1G wind dependent heat transfer for gains [W/(m²*K*m/s)]"; uc1eta0 "U1E wind dependancy of optical efficiency in W/(m²*m/s)"; hi "HI heat transfer between collector and tube [W/(m2.K)]"; c_abs "effective heat capacity of absorber [J/(m²*K)]"; c_fl "effective heat capacity of fluid [J/(m²*K)]"; lin "linear pressure drop in Pa/(kg/s)"; qua "quadratic pressure drop in Pa/(kg/s)²"; tini "initial temperature [degree centigrade]"; nodes "number of nodes (>=2)"
      mask help:
      | 2xN-nodes model:
      | c_abs*dTp/dt=qdot_solar-qdot_conv_gain-qdot_conv_loss-qdot_cond
      |             -qdot_sky-qdot_fluid
      | qdot_solar = absorbed_solar_radiation - U1E*Iglb*vwind
      | qdot_conv_gain = fconv * (U0G + U1G*vwind)*(Tp - Tamb)
      | qdot_conv_loss = (1-fconv)*(U0L + U1L*vwind)*(Tp - Tamb)
      | qdot_cond = fcond*(U0C + U1C*vwind)*ccond*(ps(Tdew) - ps(Tp))
      | qdot_sky = e * const_sigma*(Tp^4 - Tsky^4)
      | qdot_fluid = HI*(Tp-Tfluid)
      | fconv = 1 if Tp > Tamb, 0 otherwise
      | fcond = 1 if Tp below dewpoint, 0 otherwise
      | Look under mask to change the incidence angle modifier, the pressure drop and the radiation calculation method.
      mask init:
      | acol = max(acol, 0.01);
      | fta = max(fta,0);
      | inv_c_abs = 1/max(c_abs,1);
      | inv_c_fl = 1/max(c_fl,1);
      mask Help: web(fullfile(path_carnot('help'),'Collector_Unglazed.html'),'-helpbrowser')
      mask DialogControl ParameterTabVar0 Prompt: Geometry
      mask DialogControl ParameterTabVar01 Prompt: Coll.Parameters
      mask DialogControl ParameterTabVar012 Prompt: Hydraulic
      mask DialogControl ParameterTabVar0123 Prompt: Calculation
      mask Display: plot(-30,-30,130,120,[0,70,70,0,0],[-0,-0,5,5,-0],[30,30,100,100,30],[100,94,94,100,100],[32,1],[94,5],[40,10],[94,5],[49,19],[94,5],[57,27],[94,5],[65,35],[94,5],[73,43],[94,5],[82,51],[94,5],[90,60],[94,5],[98,68],[94,5])
  Divide : Product  Inputs=/*
  Gain : Gain  Gain=Ncollector
  Gain3 : Gain  Gain=Ncollector
  Ncollector : Constant  Value=Ncollector
  T_Sensor1 : $bdroot/Control/T_Sensor  tc=SensorTimeConstant  t0=tini
  Cdat : Outport
  Tsol : Outport  Port=2
  THBs : Outport  Port=3
  wires:
  T_Sensor1/2 -> Tsol/1  "Tsol"
  T_Sensor1/1 -> THBs/1  "THB_s"
  Collector_Unglazed/2(THB_s) -> Bus Assignment1/1
  WDB/1 -> Collector_Unglazed/1(WDB)
  position/1 -> Collector_Unglazed/2(position)
  THBr/1 -> Bus Assignment/1, Bus Selector/1
  Collector_Unglazed/1(Cdat) -> Bus Assignment2/1, Bus Selector1/1
  Bus Assignment/1 -> Collector_Unglazed/3(THB_r)
  Bus Assignment1/1 -> T_Sensor1/1
  Bus Selector/1 -> Divide/2, Bus Assignment2/5, Bus Assignment2/4, Bus Assignment1/2  "<MassFlow>"
  Ncollector/1 -> Divide/1
  Divide/1 -> Bus Assignment/2
  Bus Selector1/1 -> Gain/1  "<Acol>"
  Bus Selector1/2 -> Gain3/1  "<Qdot>"
  Gain/1 -> Bus Assignment2/2
  Gain3/1 -> Bus Assignment2/3
  Bus Assignment2/1 -> Cdat/1

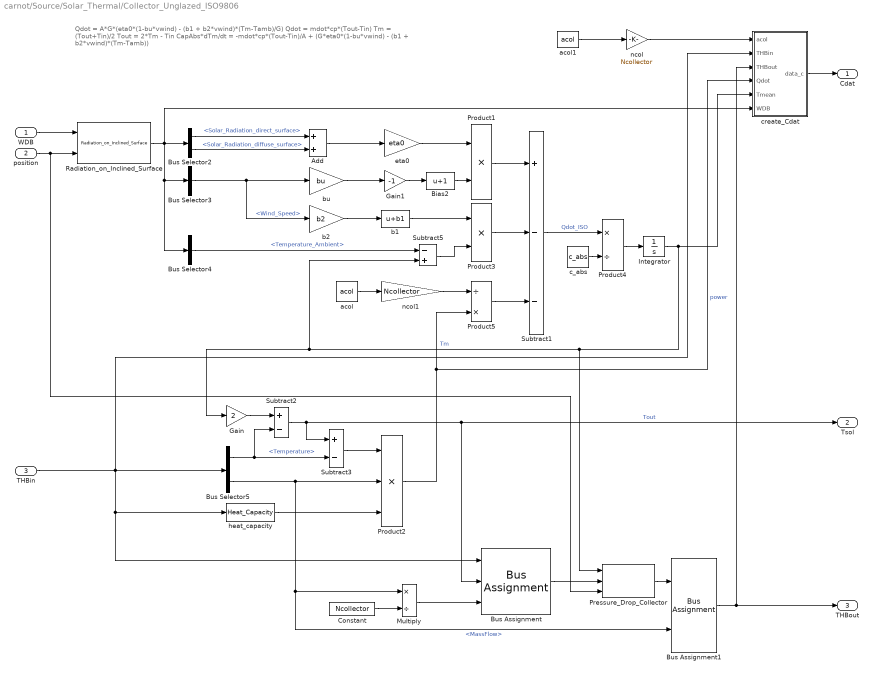
== system carnot/Source/Solar_Thermal/Collector_Unglazed_ISO9806 ==
  note: Qdot = A*G*(eta0*(1-bu*vwind) - (b1 + b2*vwind)*(Tm-Tamb)/G)
      | Qdot = mdot*cp*(Tout-Tin)
      | Tm = (Tout+Tin)/2
      | Tout = 2*Tm - Tin
      | CapAbs*dTm/dt = -mdot*cp*(Tout-Tin)/A + (G*eta0*(1-bu*vwind) - (b1 + b2*vwind)*(Tm-Tamb))
  WDB : Inport
  position : Inport  Port=2
  THBin : Inport  Port=3
  Add : Sum  Inputs=2
  Bias2 : Bias  Bias=1
  Bus Assignment : BusAssignment  AssignedSignals=Temperature,MassFlow
  Bus Assignment1 : BusAssignment  AssignedSignals=MassFlow
  Bus Selector2 : BusSelector  OutputSignals=Solar_Radiation_direct_surface,Solar_Radiation_diffuse_surface
  Bus Selector3 : BusSelector  OutputSignals=Wind_Speed
  Bus Selector4 : BusSelector  OutputSignals=Temperature_Ambient
  Bus Selector5 : BusSelector  OutputSignals=Temperature,MassFlow
  Constant : Constant  Value=Ncollector
  Gain : Gain  Gain=2
  Gain1 : Gain  Gain=-1
  Integrator : Integrator  InitialCondition=tini
  Multiply : Product  Inputs=*/
  Pressure_Drop_Collector : $bdroot/Basic/Pressure_Drop/Pressure_Drop_Collector  len=len  lin=dplin  qua=dpqua
  Product1 : Product  RndMeth=Zero
  Product2 : Product  Inputs=3  RndMeth=Zero
  Product3 : Product  RndMeth=Zero
  Product4 : Product  Inputs=*/  RndMeth=Zero
  Product5 : Product  Inputs=/*  RndMeth=Zero
  Radiation_on_Inclined_Surface : $bdroot/Weather/Radiation_on_Inclined_Surface  sky=Perez 1990  reflect=0.2
  Subtract1 : Sum  Inputs=+--
  Subtract2 : Sum  Inputs=+-
  Subtract3 : Sum  Inputs=+-
  Subtract5 : Sum  Inputs=-+
  acol : Constant  Value=acol
  acol1 : Constant  Value=acol
  b1 : Bias  Bias=b1
  b2 : Gain  Gain=b2
  bu : Gain  Gain=bu
  c_abs : Constant  Value=c_abs
  create_Cdat : Subsystem
  eta0 : Gain  Gain=eta0
  heat_capacity : $bdroot/Basic/Material_Properties/Heat_Capacity  VariantControl=CarlibClassic  INPUTARGUMENTS=THB  DEBUGLEVEL=DEBUGLEVEL  MAXTOTALWARNINGS=inf  MAXCONSECUTIVEWARNINGS=inf  WRITETOFILE=0  FILENAME='errors.txt'
  ncol : Gain  Gain=Ncollector
  ncol1 : Gain  Gain=Ncollector
  Cdat : Outport
  Tsol : Outport  Port=2
  THBout : Outport  Port=3  InitialOutput=0
  wires:
  Bus Assignment1/1 -> create_Cdat/3(THBout), THBout/1
  Multiply/1 -> Bus Assignment/3
  Constant/1 -> Multiply/2
  Integrator/1 -> create_Cdat/5(Tmean), Pressure_Drop_Collector/1, Subtract5/2, Gain/1  "Tm"
  Product1/1 -> Subtract1/1
  Bus Selector4/1 -> Subtract5/1  "<Temperature_Ambient>"
  Bus Selector2/1 -> Add/1  "<Solar_Radiation_direct_surface>"
  Bus Selector5/1 -> Subtract2/2, Subtract3/2  "<Temperature>"
  Bus Selector2/2 -> Add/2  "<Solar_Radiation_diffuse_surface>"
  heat_capacity/1 -> Product2/3
  THBin/1 -> create_Cdat/2(THBin), Bus Assignment/1, heat_capacity/1, Bus Selector5/1
  b2/1 -> b1/1
  Product3/1 -> Subtract1/2
  eta0/1 -> Product1/1
  Subtract5/1 -> Product3/2
  Bus Selector3/1 -> bu/1, b2/1  "<Wind_Speed>"
  b1/1 -> Product3/1
  Add/1 -> eta0/1
  Bias2/1 -> Product1/2
  Gain/1 -> Subtract2/1
  Radiation_on_Inclined_Surface/1 -> create_Cdat/6(WDB), Bus Selector3/1, Bus Selector4/1, Bus Selector2/1
  Product5/1 -> Subtract1/3
  Bus Selector5/2 -> Product2/2, Multiply/1, Bus Assignment1/2  "<MassFlow>"
  Subtract2/1 -> Subtract3/1, Bus Assignment/2, Tsol/1  "Tout"
  Subtract3/1 -> Product2/1
  Product2/1 -> create_Cdat/4(Qdot), Product5/2  "power"
  WDB/1 -> Radiation_on_Inclined_Surface/1
  create_Cdat/1(data_c) -> Cdat/1
  Product4/1 -> Integrator/1
  Subtract1/1 -> Product4/1  "Qdot_ISO"
  acol1/1 -> ncol/1
  position/1 -> Pressure_Drop_Collector/3, Radiation_on_Inclined_Surface/2
  c_abs/1 -> Product4/2
  acol/1 -> ncol1/1
  bu/1 -> Gain1/1
  Pressure_Drop_Collector/1 -> Bus Assignment1/1
  Bus Assignment/1 -> Pressure_Drop_Collector/2
  ncol/1 -> create_Cdat/1(acol)
  ncol1/1 -> Product5/1
  Gain1/1 -> Bias2/1

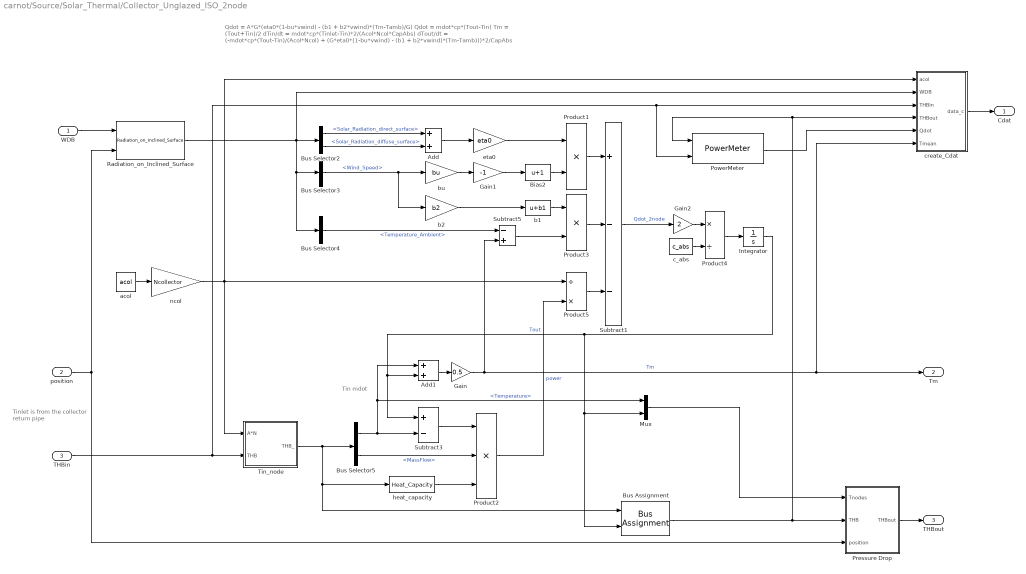
== system carnot/Source/Solar_Thermal/Collector_Unglazed_ISO_2node ==
  note: Tinlet is from the
      | collector return pipe
  note: Tin
      | mdot
  note: Qdot = A*G*(eta0*(1-bu*vwind) - (b1 + b2*vwind)*(Tm-Tamb)/G)
      | Qdot = mdot*cp*(Tout-Tin)
      | Tm = (Tout+Tin)/2
      | dTin/dt = mdot*cp*(Tinlet-Tin)*2/(Acol*Ncol*CapAbs)
      | dTout/dt = (-mdot*cp*(Tout-Tin)/(Acol*Ncol) + (G*eta0*(1-bu*vwind) - (b1 + b2*vwind)*(Tm-Tamb)))*2/CapAbs
  WDB : Inport
  position : Inport  Port=2
  THBin : Inport  Port=3
  Add : Sum  Inputs=2
  Add1 : Sum
  Bias2 : Bias  Bias=1
  Bus Assignment : BusAssignment  AssignedSignals=Temperature
  Bus Selector2 : BusSelector  OutputSignals=Solar_Radiation_direct_surface,Solar_Radiation_diffuse_surface
  Bus Selector3 : BusSelector  OutputSignals=Wind_Speed
  Bus Selector4 : BusSelector  OutputSignals=Temperature_Ambient
  Bus Selector5 : BusSelector  OutputSignals=Temperature,MassFlow
  Gain : Gain  Gain=0.5
  Gain1 : Gain  Gain=-1
  Gain2 : Gain  Gain=2
  Integrator : Integrator  InitialCondition=tini
  Mux : Mux  Inputs=2
  PowerMeter : $bdroot/Control/PowerMeter
  Pressure Drop : Subsystem
  Product1 : Product  RndMeth=Zero
  Product2 : Product  Inputs=3  RndMeth=Zero
  Product3 : Product  RndMeth=Zero
  Product4 : Product  Inputs=*/  RndMeth=Zero
  Product5 : Product  Inputs=/*  RndMeth=Zero
  Radiation_on_Inclined_Surface : $bdroot/Weather/Radiation_on_Inclined_Surface  sky=Perez 1990  reflect=0.2
  Subtract1 : Sum  Inputs=+--
  Subtract3 : Sum  Inputs=+-
  Subtract5 : Sum  Inputs=-+
  Tin_node : Subsystem
  acol : Constant  Value=acol
  b1 : Bias  Bias=b1
  b2 : Gain  Gain=b2
  bu : Gain  Gain=bu
  c_abs : Constant  Value=c_abs
  create_Cdat : Subsystem
  eta0 : Gain  Gain=eta0
  heat_capacity : $bdroot/Basic/Material_Properties/Heat_Capacity  VariantControl=CarlibClassic  INPUTARGUMENTS=THB  DEBUGLEVEL=DEBUGLEVEL  MAXTOTALWARNINGS=inf  MAXCONSECUTIVEWARNINGS=inf  WRITETOFILE=0  FILENAME='errors.txt'
  ncol : Gain  Gain=Ncollector
  Cdat : Outport
  Tm : Outport  Port=2
  THBout : Outport  Port=3  InitialOutput=0
  wires:
  PowerMeter/1 -> create_Cdat/5(Qdot)
  Gain1/1 -> Bias2/1
  ncol/1 -> Product5/1, create_Cdat/1(acol), Tin_node/1(A*N)
  Bus Assignment/1 -> PowerMeter/1, create_Cdat/4(THBout), Pressure Drop/2(THB)
  bu/1 -> Gain1/1
  acol/1 -> ncol/1
  c_abs/1 -> Product4/2
  position/1 -> Radiation_on_Inclined_Surface/2, Pressure Drop/3(position)
  Subtract1/1 -> Gain2/1  "Qdot_2node"
  Product4/1 -> Integrator/1
  create_Cdat/1(data_c) -> Cdat/1
  WDB/1 -> Radiation_on_Inclined_Surface/1
  Product2/1 -> Product5/2  "power"
  Subtract3/1 -> Product2/1
  Bus Selector5/2 -> Product2/2  "<MassFlow>"
  Product5/1 -> Subtract1/3
  Radiation_on_Inclined_Surface/1 -> create_Cdat/2(WDB), Bus Selector4/1, Bus Selector3/1, Bus Selector2/1
  Bias2/1 -> Product1/2
  Add/1 -> eta0/1
  b1/1 -> Product3/1
  Bus Selector3/1 -> b2/1, bu/1  "<Wind_Speed>"
  Subtract5/1 -> Product3/2
  eta0/1 -> Product1/1
  Product3/1 -> Subtract1/2
  b2/1 -> b1/1
  heat_capacity/1 -> Product2/3
  Bus Selector2/2 -> Add/2  "<Solar_Radiation_diffuse_surface>"
  Bus Selector5/1 -> Subtract3/2, Mux/1, Add1/1  "<Temperature>"
  Bus Selector2/1 -> Add/1  "<Solar_Radiation_direct_surface>"
  Bus Selector4/1 -> Subtract5/1  "<Temperature_Ambient>"
  Product1/1 -> Subtract1/1
  Pressure Drop/1(THBout) -> THBout/1
  Tin_node/1(THB_) -> Bus Selector5/1, heat_capacity/1, Bus Assignment/1
  THBin/1 -> create_Cdat/3(THBin), PowerMeter/2, Tin_node/2(THB)
  Integrator/1 -> Subtract3/1, Add1/2, Bus Assignment/2, Mux/2  "Tout"
  Add1/1 -> Gain/1
  Gain/1 -> Subtract5/2, create_Cdat/6(Tmean), Tm/1  "Tm"
  Mux/1 -> Pressure Drop/1(Tnodes)
  Gain2/1 -> Product4/1
